simulink model "inverted_pendulum_control"  (R2024b)
settings: Solver=VariableStepAuto  StartTime=0.0  StopTime=10  RelTol=1e-3
undefined symbols (not defined in the file): A, B, K_integral, K_states
settings Model: Creator=lenovo x390  LastModifiedBy=lenovo x390

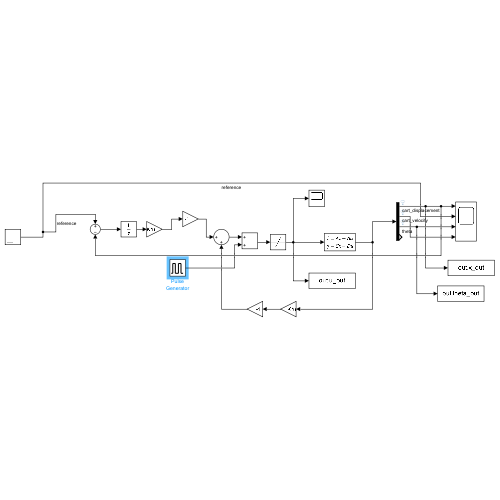
[thumbnail: Simulink's stored preview of the top-level diagram]
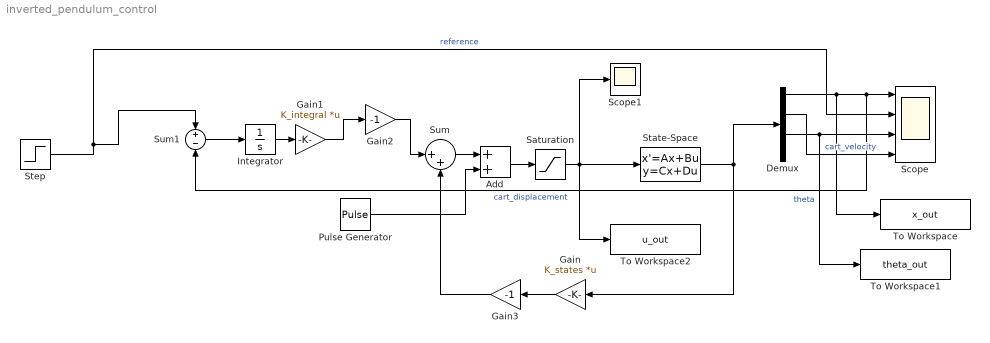
== system inverted_pendulum_control ==
  Add : Sum
  Demux : Demux
  Gain : Gain  Gain=K_states  Multiplication=Matrix(K*u)
  Gain1 : Gain  Gain=K_integral  Multiplication=Matrix(K*u)
  Gain2 : Gain  Gain=-1
  Gain3 : Gain  Gain=-1
  Integrator : Integrator
  Pulse Generator : DiscretePulseGenerator  PulseType=Time based  Amplitude=1000  Period=10  PulseWidth=0.001  PhaseDelay=1
  Saturation : Saturate  UpperLimit=10  LowerLimit=-10
  Scope : Scope  NumInputPorts=4
  Scope1 : Scope
  State-Space : StateSpace  A=A  B=B  C=eye(4)  D=zeros(4,1)  InitialCondition=0
  Step : Step  Time=0  After=5  SampleTime=0
  Sum : Sum  Inputs=|++
  Sum1 : Sum  Inputs=+-
  To Workspace : ToWorkspace  VariableName=x_out  SaveFormat=Timeseries  SampleTime=-1
  To Workspace1 : ToWorkspace  VariableName=theta_out  SaveFormat=Timeseries  SampleTime=-1
  To Workspace2 : ToWorkspace  VariableName=u_out  SaveFormat=Timeseries  SampleTime=-1
  wires:
  State-Space/1 -> Demux/1, Gain/1
  Gain1/1 -> Gain2/1
  Saturation/1 -> To Workspace2/1, Scope1/1, State-Space/1
  Demux/3 -> To Workspace1/1, Scope/3  "theta"
  Gain/1 -> Gain3/1
  Integrator/1 -> Gain1/1
  Sum/1 -> Add/1
  Add/1 -> Saturation/1
  Pulse Generator/1 -> Add/2
  Demux/1 -> To Workspace/1, Scope/1, Sum1/2  "cart_displacement"
  Sum1/1 -> Integrator/1
  Step/1 -> Scope/2, Sum1/1  "reference"
  Gain3/1 -> Sum/2
  Gain2/1 -> Sum/1
  Demux/2 -> Scope/4  "cart_velocity"
